simulink model "w2p1"  (R2020b)
settings: Solver=VariableStepAuto  StartTime=0.0  StopTime=10.0  RelTol=1e-3
settings Model: Creator=Dell  LastModifiedBy=Dell

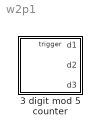
== system w2p1 ==
  3 digit mod 5 counter : Stateflow chart  TreatAsAtomicUnit=on

== stateflow chart w2p1/3 digit mod 5 counter ==
  state digit1 [parallel]
    settings: executionOrder=1
    state One
      en:
      d1=1;
    state Two
      en:
      d1=2;
    state Zero
      en:
      d1=0;
    state Three
      en:
      d1=3;
    state Four
      en:
      d1=4;
    digit1.Two -> digit1.Three : inputClick
    digit1.Zero -> digit1.One : inputClick
    digit1.One -> digit1.Two : inputClick
    (default) -> digit1.Zero
    digit1.Four -> digit1.Zero : inputClick/{digit2.in2}
    digit1.Three -> digit1.Four : inputClick
  state digit2 [parallel]
    settings: executionOrder=2
    state One
      en:
      d2=1;
    state Two
      en:
      d2=2;
    state Zero
      en:
      d2=0;
    state Three
      en:
      d2=3;
    state Four
      en:
      d2=4;
    digit2.Two -> digit2.Three : in2
    digit2.Zero -> digit2.One : in2
    digit2.One -> digit2.Two : in2
    (default) -> digit2.Zero
    digit2.Four -> digit2.Zero : in2/{digit3.in3}
    digit2.Three -> digit2.Four : in2
  state digit3 [parallel]
    settings: executionOrder=3
    state One
      en:
      d3=1;
    state Two
      en:
      d3=2;
    state Zero
      en:
      d3=0;
    state Three
      en:
      d3=3;
    state Four
      en:
      d3=4;
    digit3.Two -> digit3.Three : in3
    digit3.Zero -> digit3.One : in3
    digit3.One -> digit3.Two : in3
    (default) -> digit3.Zero
    digit3.Four -> digit3.Zero : in3
    digit3.Three -> digit3.Four : in3
  data: d1 output; d2 output; d3 output
  events: in2 local FUNCTION_CALL_EVENT; in3 local FUNCTION_CALL_EVENT; inputClick input FUNCTION_CALL_EVENT
